simulink model "TST_InnerTransition"  (Simulink 10.0)
settings: Solver=FixedStepDiscrete  StartTime=0.0  StopTime=10.0  FixedStep=0.02  RelTol=1e-3  EnableMultiTasking=on
settings Model: Creator=kharthforeign  LastModifiedBy=unknown
settings DataIOCC: LimitDataPoints=on  SignalLoggingSaveFormat=ModelDataLogs  SaveOutput=off  SignalLogging=off  SaveTime=off
settings OptimizationCC: BlockReduction=off  ConditionallyExecuteInputs=off  OptimizeBlockIOStorage=off  BufferReuse=off  GlobalBufferReuse=off  ExpressionFolding=off  ExpressionDepthLimit=2147483647  LocalBlockOutputs=off  InitFltsAndDblsToZero=on  OptimizeDataStoreBuffers=off  BusAssignmentInplaceUpdate=off
settings DebuggingCC: SolverPrmCheckMsg=warning  FcnCallInpInsideContextMsg=warning  StateNameClashWarn=warning
settings SFSimCC: SimParseCustomCode=off
settings GRTTargetCC: GeneratePreprocessorConditionals=Disable all
settings ConfigComp: CovExternalEMLEnable=off

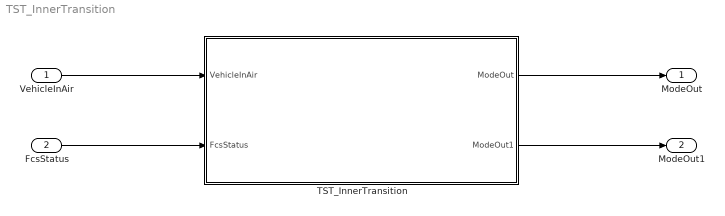
== system TST_InnerTransition ==
  VehicleInAir : Inport  OutDataTypeStr=boolean  PortDimensions=1
  FcsStatus : Inport  Port=2  OutDataTypeStr=Bus: FCS_FlightControlSystem_Status
  TST_InnerTransition : Subsystem  TreatAsAtomicUnit=on
  ModeOut : Outport  OutDataTypeStr=uint32  PortDimensions=1
  ModeOut1 : Outport  Port=2  OutDataTypeStr=uint32  PortDimensions=1
  wires:
  VehicleInAir/1 -> TST_InnerTransition/1(VehicleInAir)
  FcsStatus/1 -> TST_InnerTransition/2(FcsStatus)
  TST_InnerTransition/1(ModeOut) -> ModeOut/1
  TST_InnerTransition/2(ModeOut1) -> ModeOut1/1

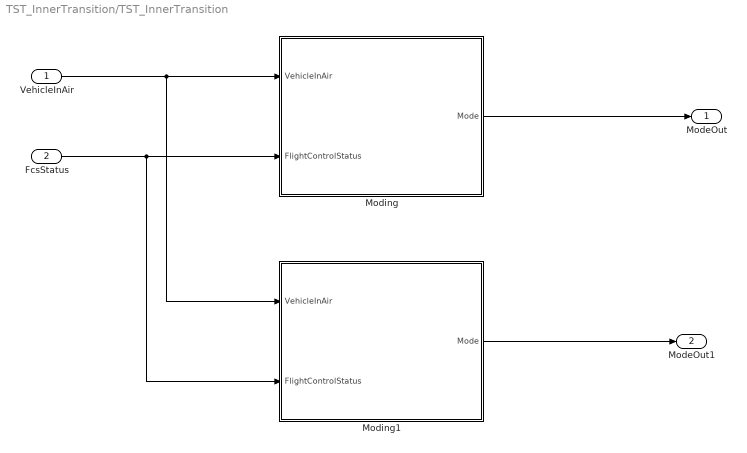
== system TST_InnerTransition/TST_InnerTransition ==
  VehicleInAir : Inport  OutDataTypeStr=boolean  PortDimensions=1
  FcsStatus : Inport  Port=2  OutDataTypeStr=Bus: FCS_FlightControlSystem_Status
  Moding : Stateflow chart  TreatAsAtomicUnit=on
  Moding1 : Stateflow chart  TreatAsAtomicUnit=on
  ModeOut : Outport  OutDataTypeStr=uint32  PortDimensions=1
  ModeOut1 : Outport  Port=2  OutDataTypeStr=uint32  PortDimensions=1
  wires:
  FcsStatus/1 -> Moding/2(FlightControlStatus), Moding1/2(FlightControlStatus)
  VehicleInAir/1 -> Moding/1(VehicleInAir), Moding1/1(VehicleInAir)
  Moding/1(Mode) -> ModeOut/1
  Moding1/1(Mode) -> ModeOut1/1

== stateflow chart TST_InnerTransition/Moding ==
  state Main
    state Off
      entry:
      Mode = uint32(1);
    state Launch
      entry:
      Mode = uint32(2);
    state Autoland
      entry:
      Mode = uint32(3);
    Main -> (junction 8) : [true]
    (default) -> Off : {UpdateFeedthroughParameters();}
    (junction 8) -> Off [order 1] : [(FlightControlStatus.PressureAltitude_Ft < 500.0) && (~VehicleInAir)]
    (junction 8) -> (junction 9) [order 2]
    (junction 9) -> Launch [order 1] : [(FlightControlStatus.PressureAltitude_Ft > 1500.0) || VehicleInAir]
    (junction 9) -> (junction 10) [order 2]
    (junction 10) -> Autoland : [(FlightControlStatus.PressureAltitude_Ft > 2500.0) || ...
        | FlightControlStatus.LeftEngFailed]
  state UpdateFeedthroughParameters [function]
    (default) -> (junction 18) : {...
        |    Mode = uint32(5);...
        | }
  (default) -> Main
  data: VehicleInAir input boolean; Mode output uint32; FlightControlStatus input FCS_FlightControlSystem_Status

== stateflow chart TST_InnerTransition/Moding1 ==
  state Main
    state Off
      entry:
      Mode = uint32(1);
    state Launch
      entry:
      Mode = uint32(2);
    state Autoland
      entry:
      Mode = uint32(3);
    (default) -> Off : {UpdateFeedthroughParameters();}
    Main -> Off [order 1] : [(FlightControlStatus.PressureAltitude_Ft < 500.0) && (~VehicleInAir)]
    Main -> Launch [order 2] : [(FlightControlStatus.PressureAltitude_Ft > 1500.0) || VehicleInAir]
    Main -> Autoland [order 3] : [(FlightControlStatus.PressureAltitude_Ft > 2500.0) || ...
        | FlightControlStatus.LeftEngFailed]
  state UpdateFeedthroughParameters [function]
    (default) -> (junction 35) : {...
        |    Mode = uint32(5);...
        | }
  (default) -> Main
  data: VehicleInAir input boolean; Mode output uint32; FlightControlStatus input FCS_FlightControlSystem_Status
